simulink model "longitunal_DynamicModel"  (R2024b)
settings: Solver=VariableStepAuto  StartTime=0.0  StopTime=4.5  MaxStep=0.001  RelTol=1e-3
undefined symbols (not defined in the file or in its folder): car
libraries: slpidlib x1, simulink x1
settings Model: Creator=greg  LastModifiedBy=franc

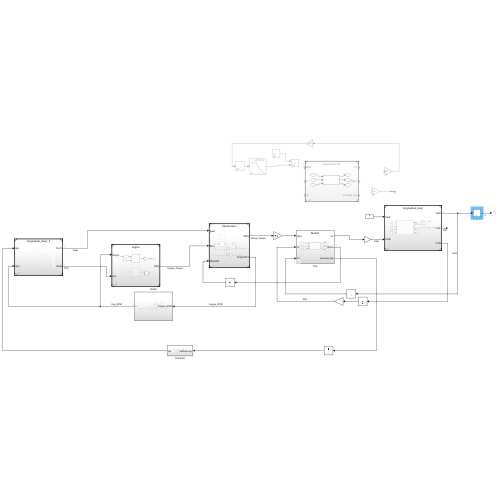
[thumbnail: Simulink's stored preview of the top-level diagram]
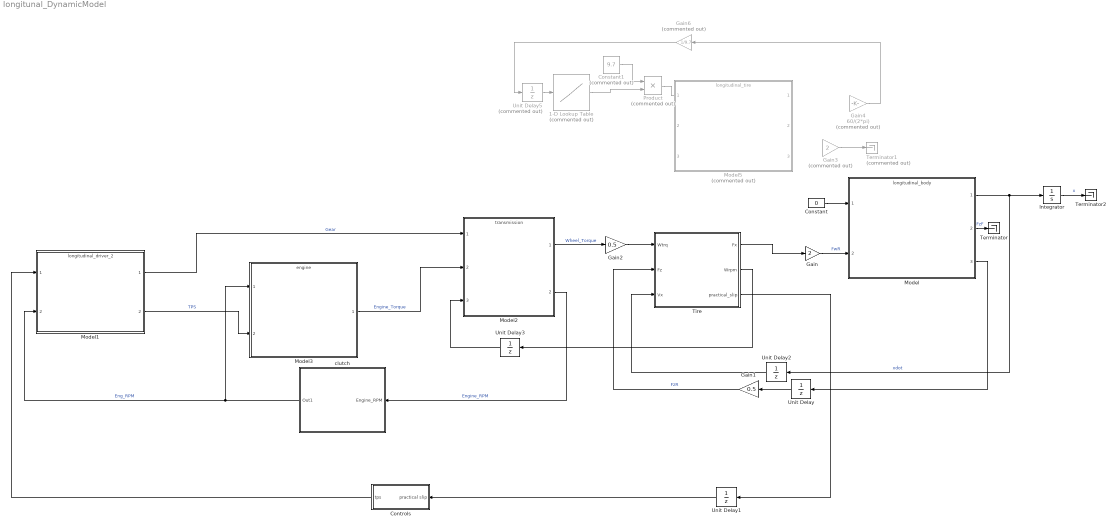
== system longitunal_DynamicModel ==
  1-D Lookup Table : Lookup_n-D  Commented=on  NumberOfTableDimensions=1  BreakpointsForDimension1=[0;5000;8000;10000;16000]  Table=[14;14;9;6;2]  InternalRulePriority=Speed  RndMeth=Simplest
  Constant : Constant  Value=0
  Constant1 : Constant  Commented=on  Value=9.7
  Controls : Subsystem
  Gain : Gain  Gain=2
  Gain1 : Gain  Gain=0.5
  Gain2 : Gain  Gain=0.5
  Gain3 : Gain  Commented=on  Gain=2
  Gain4 : Gain  Commented=on  Gain=60/(2*pi)
  Gain6 : Gain  Commented=on  Gain=1/9.7
  Integrator : Integrator
  Model : ModelReference  ModelNameDialog=longitudinal_body.slx  SimulationMode=Normal  ModelReferenceVersion=1.24
  Model1 : ModelReference  ModelNameDialog=longitudinal_driver_2.slx  SimulationMode=Normal  ModelReferenceVersion=1.10
  Model2 : ModelReference  ModelNameDialog=transmission.slx  SimulationMode=Normal  ModelReferenceVersion=1.12
  Model3 : ModelReference  ModelNameDialog=engine.slx  SimulationMode=Normal  ModelReferenceVersion=1.18
  Model5 : ModelReference  Commented=on  ModelNameDialog=longitudinal_tire.slx  SimulationMode=Normal  ModelReferenceVersion=3.7
  Product : Product  Commented=on
  Terminator : Terminator
  Terminator1 : Terminator  Commented=on
  Terminator2 : Terminator
  Tire : Subsystem  Variant=on
  Unit Delay : UnitDelay  InitialCondition=car.initialconditions.FzR  SampleTime=-1  HasFrameUpgradeWarning=on
  Unit Delay1 : UnitDelay  SampleTime=-1  HasFrameUpgradeWarning=on
  Unit Delay2 : UnitDelay  InitialCondition=car.initialconditions.xdot  SampleTime=-1  HasFrameUpgradeWarning=on
  Unit Delay3 : UnitDelay  InitialCondition=car.initialconditions.Wrpm  SampleTime=-1  HasFrameUpgradeWarning=on
  Unit Delay5 : UnitDelay  Commented=on  SampleTime=-1  HasFrameUpgradeWarning=on
  clutch : Subsystem
  wires:
  Model1/2 -> Model3/2  "TPS"
  Model1/1 -> Model2/1  "Gear"
  Model/3 -> Unit Delay/1
  Model/1 -> Integrator/1, Unit Delay2/1  "xdot"
  Unit Delay/1 -> Gain1/1
  Unit Delay2/1 -> Tire/3(Vx)
  Model3/1 -> Model2/2  "Engine_Torque"
  Model2/1 -> Gain2/1  "Wheel_Torque"
  Unit Delay3/1 -> Model2/3
  Gain/1 -> Model/2  "FwR"
  Gain1/1 -> Tire/2(Fz)  "FzR"
  Gain2/1 -> Tire/1(Wtrq)
  Model/2 -> Terminator/1  "FzF"
  Constant1/1 -> Product/1
  1-D Lookup Table/1 -> Product/2
  Product/1 -> ?
  Gain4/1 -> Gain6/1
  Gain6/1 -> Unit Delay5/1
  Unit Delay5/1 -> 1-D Lookup Table/1
  Gain3/1 -> Terminator1/1
  Constant/1 -> Model/1
  Tire/2(Wrpm) -> Unit Delay3/1
  Tire/1(Fx) -> Gain/1
  Tire/3(practical_slip) -> Unit Delay1/1
  Controls/1(tps) -> Model1/1
  Unit Delay1/1 -> Controls/1(practical slip)
  Model2/2 -> clutch/1(Engine_RPM)  "Engine_RPM"
  clutch/1(Out1) -> Model1/2, Model3/1  "Eng_RPM"
  Integrator/1 -> Terminator2/1  "x"

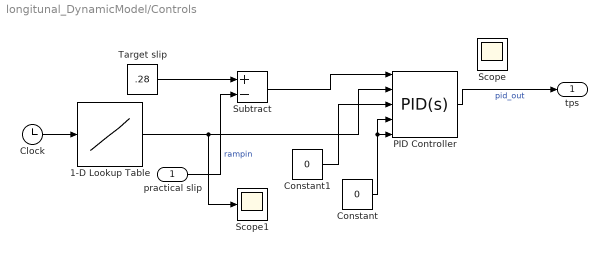
== system longitunal_DynamicModel/Controls ==
  practical slip : Inport
  1-D Lookup Table : Lookup_n-D  NumberOfTableDimensions=1  BreakpointsForDimension1=[0;0.10000000000000001;0.20000000000000001;0.29999999999999999;0.40000000000000002;0.5;0.59999999999999998;0.75;0.80000000000000004;0.90000000000000002;1;1.2]  Table=[1.5;4;10;15;18;19;20;16;18;20;25;30]  InternalRulePriority=Speed  RndMeth=Simplest
  Clock : Clock
  Constant : Constant  Value=0
  Constant1 : Constant  Value=0
  PID Controller : slpidlib/PID Controller  Controller=PID  Form=Parallel  TimeDomain=Continuous-time  UseExternalTs=off  SampleTime=-1  IntegratorMethod=Forward Euler  FilterMethod=Forward Euler  ControllerParametersSource=external  P=1.5  I=0  UseKiTs=off  D=0  UseExternalDerivativeSource=off  N=0  UseFilter=on  TunerSelectOption=Transfer Function Based (PID Tuner App)  InitialConditionSource=internal  InitialConditionForIntegrator=0  InitialConditionForFilter=0  DifferentiatorICPrevScaledInput=0  ExternalReset=none  TrackingMode=off  Kt=1  LimitOutput=on  SatLimitsSource=internal  UpperSaturationLimit=1  LowerSaturationLimit=0  LinearizeAsGain=on  AntiWindupMode=none  Kb=1  LimitIntegrator=off  UpperIntegratorSaturationLimit=inf  LowerIntegratorSaturationLimit=-inf  POutMin=[]  POutMax=[]  IOutMin=[]  IOutMax=[]  DOutMin=[]  DOutMax=[]  NOutMin=[]  NOutMax=[]  SumOutMin=[]  SumOutMax=[]  SaturationOutMin=[]  SaturationOutMax=[]  PParamMin=[]  PParamMax=[]  IParamMin=[]  IParamMax=[]  DParamMin=[]  DParamMax=[]  NParamMin=[]  NParamMax=[]  KbParamMin=[]  KbParamMax=[]  KtParamMin=[]  KtParamMax=[]  KbOutMin=[]  KbOutMax=[]  KtOutMin=[]  KtOutMax=[]  IntegratorOutMin=[]  IntegratorOutMax=[]  FilterOutMin=[]  FilterOutMax=[]  SumI1OutMin=[]  SumI1OutMax=[]  SumI2OutMin=[]  SumI2OutMax=[]  SumI3OutMin=[]  SumI3OutMax=[]  SumI4OutMin=[]  SumI4OutMax=[]  SumDOutMin=[]  SumDOutMax=[]  DifferentiatorOutMin=[]  DifferentiatorOutMax=[]  FilterDiffOutCoefMin=[]  FilterDiffOutCoefMax=[]  ReciprocalOutMin=[]  ReciprocalOutMax=[]  SumDenOutMin=[]  SumDenOutMax=[]  SumNumOutMin=[]  SumNumOutMax=[]  DivideOutMin=[]  DivideOutMax=[]  UdiffTsProdOutMin=[]  UdiffTsProdOutMax=[]  NTsProdOutMin=[]  NTsProdOutMax=[]  UintegralTsProdOutMin=[]  UintegralTsProdOutMax=[]  UngainTsProdOutMin=[]  UngainTsProdOutMax=[]  ClampingZeroOutDataTypeStr=Inherit: Inherit via back propagation  ClampingZeroOutMin=[]  ClampingZeroOutMax=[]  FilterDenConstantOutDataTypeStr=Inherit: Inherit via back propagation  FilterDenConstantOutMin=[]  FilterDenConstantOutMax=[]  PCopyOutDataTypeStr=Inherit: Inherit via back propagation  PCopyOutMin=[]  PCopyOutMax=[]  NCopyOutDataTypeStr=Inherit: Inherit via back propagation  NCopyOutMin=[]  NCopyOutMax=[]  IntegratorContinuousStateAttributes=''  IntegratorStateMustResolveToSignalObject=off  IntegratorRTWStateStorageClass=Auto  FilterContinuousStateAttributes=''  FilterStateMustResolveToSignalObject=off  FilterRTWStateStorageClass=Auto  ParallelPVariant=ExternalParameters  IdealPVariant=Disabled  IVariant=ExternalParameters  DVariant=ExternalParameters  IntegratorVariant=Continuous  SatVariant=Enabled  AWVariant=Passthrough  PCopyVariant=Disabled  TRVariant=Disabled  FdbkBlocksVariant=Forward  IdealPFdbkVariant=Disabled  SatFdbkVariant=Disabled  DerivativeFilterVariant=ContFilter  NVariant=ExternalParameters  NCopyVariant=Disabled  FilterICVariant=InternalICsFilter  IntegratorICVariant=InternalICs  ExternalResetVariant=Disabled  TRSumVariant=Passthrough  SumFdbkVariant=Disabled  SumVariant=Sum_PID  TsampFilterVariant=InternalTs  TsampNgainVariant=Passthrough  TsampIntegralVariant=Disabled_SignalSpec  ExternalSaturationOutDataTypeStr=Inherit: Same as second input  DerivativeSourceVariant=ErrorSignal  PreIntVariant=InternalPreInt
  Scope : Scope
  Scope1 : Scope
  Subtract : Sum  Inputs=+-
  Target slip : Constant  Value=.28
  tps : Outport
  wires:
  practical slip/1 -> Subtract/2  "rampin"
  Target slip/1 -> Subtract/1
  Subtract/1 -> PID Controller/1
  PID Controller/1 -> tps/1  "pid_out"
  Constant/1 -> PID Controller/4, PID Controller/5
  Constant1/1 -> PID Controller/3
  Clock/1 -> 1-D Lookup Table/1
  1-D Lookup Table/1 -> PID Controller/2, Scope1/1

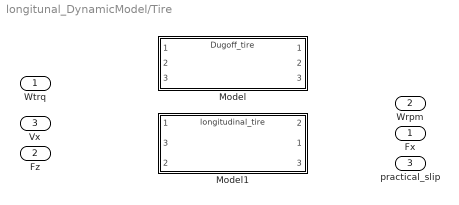
== system longitunal_DynamicModel/Tire ==
  Wtrq : Inport
  Fz : Inport  Port=2
  Vx : Inport  Port=3
  Model : ModelReference  DisableCoverage=on  ModelNameDialog=Dugoff_tire.slx  SimulationMode=Normal  VariantControl=false  ModelReferenceVersion=2.16
  Model1 : ModelReference  ModelNameDialog=longitudinal_tire.slx  SimulationMode=Normal  VariantControl=true  ModelReferenceVersion=3.7
      settings: PortSchema="{\"entries\":[{\"content\":{\"sides\":[{\"content\":{\"connectorIds\":[\"In1\",\"In3\",\"In2\"]},\"type\":\"ConnectorPlacement.EquallySpacedRectSide\",\"uuid\":\"5eba1a74-bd07-49e9-ac91-356b950fcd72\"},{\"content\":{\"connectorIds\":[\"Out2\",\"Out1\",\"Out3\"],\"side\":\"RIGHT\"},\"type\":\"ConnectorPlacement.EquallySpacedRectSide\",\"uuid\":\"1040ce78-c535-419a-aa8f-ad6fbf19e979\"},{\"content\":{\"side\":\"TOP\"},\"type\":\"ConnectorPlacement.EquallySpacedRectSide\",\"uuid\":\"ba0f3e1f-76c3-4461-91cd-c7f47b575855\"}]},\"type\":\"ConnectorPlacement.EquallySpacedConnector\",\"uuid\":\"77c71335-a5e7-4e66-a78b-88921c7c7d22\"}],\"packageUris\":[\"http://schema.mathworks.com/mf0/Connector/R2020b\"],\"version\":\"1.0\"}"
  Fx : Outport
  Wrpm : Outport  Port=2
  practical_slip : Outport  Port=3

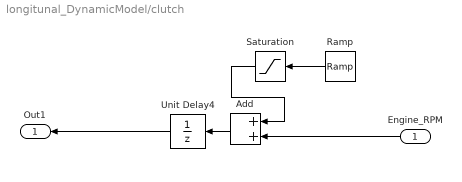
== system longitunal_DynamicModel/clutch ==
  Engine_RPM : Inport
  Add : Sum
  Ramp : simulink/Sources/Ramp  slope=-car.clutch.RPM.start/car.clutch.time.engaged  start=0  InitialOutput=car.clutch.RPM.start
  Saturation : Saturate  UpperLimit=car.initialconditions.EngineRPM  LowerLimit=0
  Unit Delay4 : UnitDelay  InitialCondition=car.initialconditions.EngineRPM  SampleTime=-1  HasFrameUpgradeWarning=on
  Out1 : Outport
  wires:
  Add/1 -> Unit Delay4/1
  Saturation/1 -> Add/1
  Ramp/1 -> Saturation/1
  Engine_RPM/1 -> Add/2
  Unit Delay4/1 -> Out1/1
